simulink model "Espacio_Estados_sin_ROS_Trayectorias"  (R2023a)
settings: Solver=FixedStepAuto  StartTime=0.0  StopTime=t_final  FixedStep=T  RelTol=1e-3
undefined symbols (not defined in the file): A, B, C, D, Ke, Ki, T
libraries: robotcorelib x1
settings Model: Creator=mluser  LastModifiedBy=camarin
settings SolverCC: AlgebraicLoopSolver=TrustRegion
settings DataIOCC: ReturnWorkspaceOutputs=off
settings DebuggingCC: UnconnectedInputMsg=warning  UnconnectedOutputMsg=warning  UnconnectedLineMsg=warning
settings ModelReferenceCC: EnableRefExpFcnMdlSchedulingChecks=on
settings RTWCC: DLArmComputeVersion=19.05

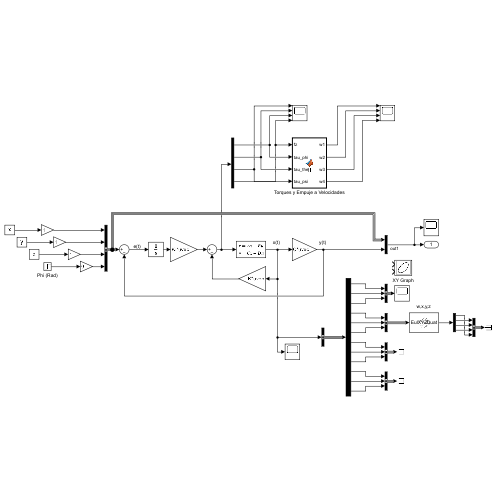
[thumbnail: Simulink's stored preview of the top-level diagram]
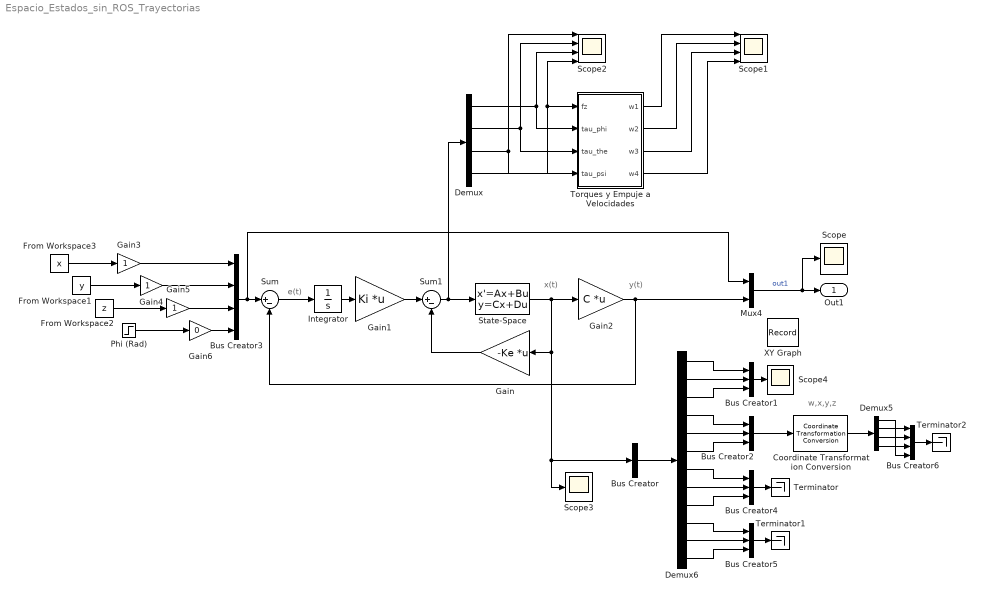
== system Espacio_Estados_sin_ROS_Trayectorias ==
  note: e(t)
  note: y(t)
  note: x(t)
  note: w,x,y,z
  Bus Creator : BusCreator  Inputs=1
  Bus Creator{1..2,4..5} (4 alike) : BusCreator  Inputs=3
  Bus Creator3 : BusCreator  Inputs=4
  Bus Creator6 : BusCreator  Inputs=4
  Coordinate Transformation Conversion : robotcorelib/Coordinate Transformation Conversion  InputRepresentation=Euler Angles  InputEulerSequence=XYZ  ShowTrVecInputPort=on  OutputRepresentation=Quaternion  OutputEulerSequence=ZYX  ShowTrVecOutputPort=on  SimulateUsing=Interpreted execution
  Demux : Demux
  Demux5 : Demux
  Demux6 : Demux  Outputs=12
  From Workspace1 : FromWorkspace  VariableName=y  OutDataTypeStr=double  SampleTime=-1
  From Workspace2 : FromWorkspace  VariableName=z  OutDataTypeStr=double  SampleTime=-1
  From Workspace3 : FromWorkspace  VariableName=x  OutDataTypeStr=double  SampleTime=-1
  Gain : Gain  Gain=-Ke  Multiplication=Matrix(K*u) (u vector)
  Gain1 : Gain  Gain=Ki  Multiplication=Matrix(K*u) (u vector)
  Gain2 : Gain  Gain=C  Multiplication=Matrix(K*u) (u vector)
  Gain3 : Gain
  Gain4 : Gain
  Gain5 : Gain
  Gain6 : Gain  Gain=0
  Integrator : Integrator
  Mux4 : Mux  Inputs=2
  Phi (Rad) : Step  Time=3  SampleTime=T
  Scope : Scope
  Scope1 : Scope  NumInputPorts=4
  Scope2 : Scope  NumInputPorts=4
  Scope3 : Scope
  Scope4 : Scope
  State-Space : StateSpace  A=A  B=B  C=eye(12)  D=D  InitialCondition=0  ParameterTunability=Unconstrained
  Sum : Sum  Inputs=|+-
  Sum1 : Sum  Inputs=|+-
  Terminator : Terminator
  Terminator1 : Terminator
  Terminator2 : Terminator
  Torques y Empuje a Velocidades : MATLAB Function  TreatAsAtomicUnit=on
  XY Graph : Record  FileSettingsInternal="{\"entries\":[{\"content\":{\"excelSettings\":{\"content\":{},\"type\":\"Streamout.ExcelSettings\"}},\"type\":\"Streamout.FileSettingStorage\",\"uuid\":\"\"}],\"packageUris\":[\"http:\\/\\/schema.mathworks.com\\/mf0\\/streamout_blocks\\/R2020a\"],\"version\":\"1.0\"}"  Layout=[1 1]  SignalsInternal="{\"entries\":[{\"content\":{\"signals\":[{\"content\":{\"blockPath\":[],\"dimensions\":[1],\"domain\":\"\",\"lineColor\":\"#a2142f\",\"plots\":[1],\"port\":1,\"sid\":[\"\"],\"signalID\":5879,\"signalName\":\"Demux6:1\"},\"type\":\"RecordBlkView.Signal\",\"uuid\":\"\"},{\"content\":{\"blockPath\":[],\"dimensions\":[1],\"domain\":\"\",\"lineColor\":\"#139fff\",\"plots\":[1],\"port\":2,\"sid\":[\"\"],\"signalID\":5883,\"signalName\":\"Demux6:2\"},\"type\":\"RecordBlkView.Signal\",\"uuid\":\"\"}]},\"type\":\"RecordBlkView.InputSignals\",\"uuid\":\"\"}],\"packageUris\":[\"http:\\/\\/schema.mathworks.com\\/mf0\\/streamout_blocks\\/R2020a\"],\"version\":\"1.0\"}"  VisualizationBindings="{\"xyplotplugin\":{\"info\":[{\"series\":[{\"bindingParametersList\":[{\"parameter\":\"X-Axis\",\"signalID\":5879,\"signalName\":\"Demux6:1\"},{\"parameter\":\"Y-Axis\",\"signalID\":5883,\"signalName\":\"Demux6:2\"}],\"seriesID\":8683}],\"subplotID\":1}]}}"  CompatibilityTag=XY
  Out1 : Outport
  wires:
  State-Space/1 -> Gain2/1, Scope3/1, Bus Creator/1, Gain/1
  Mux4/1 -> Scope/1, Out1/1  "out1"
  Bus Creator3/1 -> Sum/1, Mux4/1
  Phi (Rad)/1 -> Gain6/1
  Sum/1 -> Integrator/1
  Sum1/1 -> Demux/1, State-Space/1
  Gain2/1 -> Mux4/2, Sum/2
  Gain/1 -> Sum1/2
  Integrator/1 -> Gain1/1
  Gain1/1 -> Sum1/1
  Torques y Empuje a Velocidades/1(w1) -> Scope1/1
  Torques y Empuje a Velocidades/2(w2) -> Scope1/2
  Torques y Empuje a Velocidades/3(w3) -> Scope1/3
  Torques y Empuje a Velocidades/4(w4) -> Scope1/4
  Demux/1 -> Scope2/3, Torques y Empuje a Velocidades/2(tau_phi)
  Demux/2 -> Scope2/2, Torques y Empuje a Velocidades/3(tau_the)
  Demux/3 -> Scope2/1, Torques y Empuje a Velocidades/4(tau_psi)
  Demux/4 -> Scope2/4, Torques y Empuje a Velocidades/1(fz)
  Demux6/1 -> Bus Creator1/1
  Demux6/2 -> Bus Creator1/2
  Demux6/3 -> Bus Creator1/3
  Demux6/4 -> Bus Creator2/1
  Demux6/5 -> Bus Creator2/2
  Demux6/6 -> Bus Creator2/3
  Demux6/7 -> Bus Creator4/1
  Demux6/8 -> Bus Creator4/2
  Demux6/9 -> Bus Creator4/3
  Demux6/10 -> Bus Creator5/1
  Demux6/11 -> Bus Creator5/2
  Demux6/12 -> Bus Creator5/3
  Demux5/2 -> Bus Creator6/1
  Bus Creator2/1 -> Coordinate Transformation Conversion/1
  Demux5/3 -> Bus Creator6/2
  Demux5/4 -> Bus Creator6/3
  Demux5/1 -> Bus Creator6/4
  Coordinate Transformation Conversion/1 -> Demux5/1
  Bus Creator/1 -> Demux6/1
  Gain3/1 -> Bus Creator3/1
  Gain4/1 -> Bus Creator3/2
  Gain5/1 -> Bus Creator3/3
  Gain6/1 -> Bus Creator3/4
  From Workspace3/1 -> Gain3/1
  From Workspace1/1 -> Gain4/1
  From Workspace2/1 -> Gain5/1
  Bus Creator4/1 -> Terminator/1
  Bus Creator5/1 -> Terminator1/1
  Bus Creator6/1 -> Terminator2/1
  Bus Creator1/1 -> Scope4/1

== matlab function Espacio_Estados_sin_ROS_Trayectorias/Torques y Empuje a Velocidades ==
  data: fz input; w1 output; tau_phi input; w2 output; w3 output; w4 output; tau_the input; tau_psi input
function [w1,w2,w3,w4] = H(fz,tau_phi,tau_the,tau_psi)
%         Salidas          Entradas

% Constantes 
l = 0.2;    % m
kf = 0.007; % Nm/A
km = 0.8;   % V/kRPM

% Matriz H
H = [kf     kf      kf      kf;
     0      l*kf    0       -l*kf;
     -l*kf  0       l*kf    0;  
     km     -km     km      -km];
 
% Inversa de H
H_inversa = inv(H);

% Vector de entrada
Torques = [fz;
           tau_phi;
           tau_the;
           tau_psi];
       
% Vector de salida      
Wi2 = H_inversa * Torques;


% Velocidades angulares al cuadrado
w1 = sqrt(abs(Wi2(1))) + 25;
w2 = sqrt(abs(Wi2(2))) + 25;
w3 = sqrt(abs(Wi2(3))) + 25;
w4 = sqrt(abs(Wi2(4))) + 25;


% Saturación de las velocidades angulares
RPM = 1020;
wmax = RPM*2*pi/60;
if w1>wmax
    w1 = wmax;
end
if w2>wmax
    w2 = wmax;
end
if w3>wmax
    w3 = wmax;
end
if w4>wmax
    w4 = wmax;
end
